simulink model "Question5"  (R2023b)
settings: Solver=VariableStepAuto  StartTime=0.0  StopTime=10.0  RelTol=1e-3
settings Model: Creator=akank  LastModifiedBy=akank

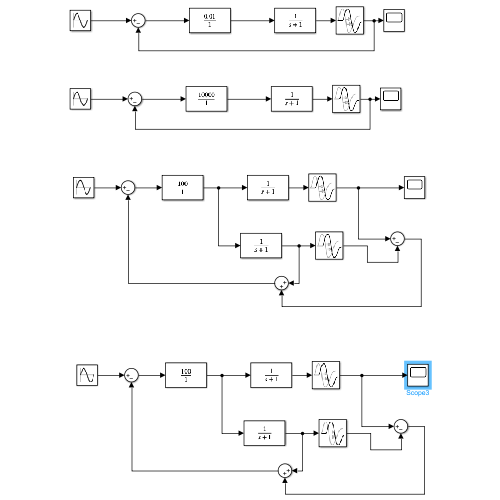
[thumbnail: Simulink's stored preview of the top-level diagram]
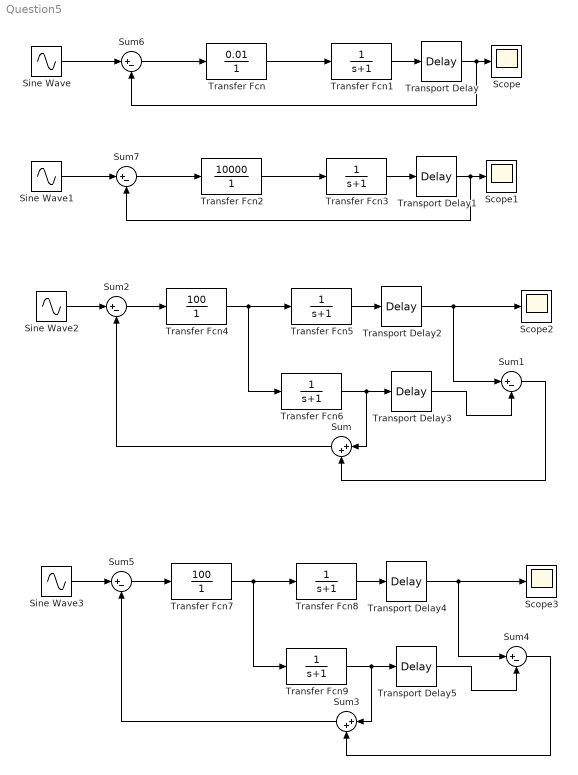
== system Question5 ==
  Scope{,1..3} (4 alike) : Scope
  Sine Wave{,1..3} (4 alike) : Sin  Frequency=120  SampleTime=0
  Sum : Sum  Inputs=|++
  Sum{1..2,4..7} (6 alike) : Sum  Inputs=|+-
  Sum3 : Sum  Inputs=|++
  Transfer Fcn : TransferFcn  Numerator=[0.01]  Denominator=[1]
  Transfer Fcn{1,3,5..6,8..9} (6 alike) : TransferFcn  Denominator=[1 1]
  Transfer Fcn2 : TransferFcn  Numerator=[10000]  Denominator=[1]
  Transfer Fcn4 : TransferFcn  Numerator=[100]  Denominator=[1]
  Transfer Fcn7 : TransferFcn  Numerator=[100]  Denominator=[1]
  Transport Delay{,1..3} (4 alike) : TransportDelay  DelayTime=0.5
  Transport Delay4 : TransportDelay  DelayTime=0.0005
  Transport Delay5 : TransportDelay  DelayTime=0.0005
  wires:
  Sum2/1 -> Transfer Fcn4/1
  Transfer Fcn/1 -> Transfer Fcn1/1
  Transfer Fcn7/1 -> Transfer Fcn9/1, Transfer Fcn8/1
  Transfer Fcn3/1 -> Transport Delay1/1
  Transfer Fcn8/1 -> Transport Delay4/1
  Transfer Fcn9/1 -> Sum3/1, Transport Delay5/1
  Sum6/1 -> Transfer Fcn/1
  Sum4/1 -> Sum3/2
  Transport Delay5/1 -> Sum4/2
  Sine Wave1/1 -> Sum7/1
  Sine Wave/1 -> Sum6/1
  Transport Delay4/1 -> Sum4/1, Scope3/1
  Sum1/1 -> Sum/2
  Transfer Fcn1/1 -> Transport Delay/1
  Transport Delay3/1 -> Sum1/2
  Sum7/1 -> Transfer Fcn2/1
  Sine Wave2/1 -> Sum2/1
  Sine Wave3/1 -> Sum5/1
  Transfer Fcn6/1 -> Sum/1, Transport Delay3/1
  Sum/1 -> Sum2/2
  Transfer Fcn2/1 -> Transfer Fcn3/1
  Transport Delay2/1 -> Sum1/1, Scope2/1
  Transport Delay1/1 -> Sum7/2, Scope1/1
  Sum3/1 -> Sum5/2
  Transfer Fcn5/1 -> Transport Delay2/1
  Transfer Fcn4/1 -> Transfer Fcn6/1, Transfer Fcn5/1
  Sum5/1 -> Transfer Fcn7/1
  Transport Delay/1 -> Sum6/2, Scope/1
